simulink model "p2c1"  (R2023b)
settings: Solver=VariableStepAuto  StartTime=0.0  StopTime=100  RelTol=1e-3
settings Model: Creator=tanvi  LastModifiedBy=tanvi

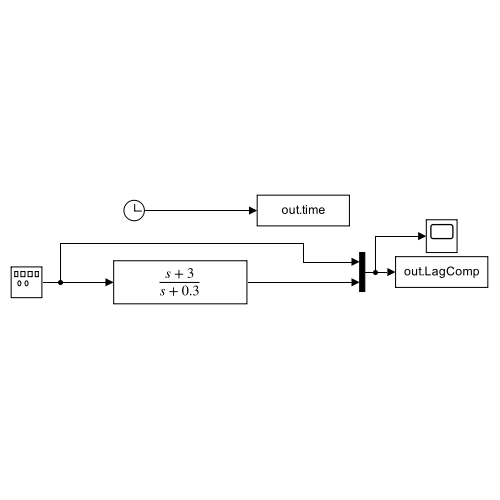
[thumbnail: Simulink's stored preview of the top-level diagram]
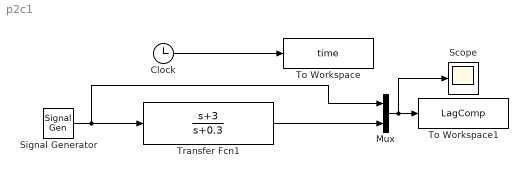
== system p2c1 ==
  Clock : Clock
  Mux : Mux  Inputs=2
  Scope : Scope
  Signal Generator : SignalGenerator  WaveForm=square  Frequency=0.02
  To Workspace : ToWorkspace  VariableName=time  SampleTime=-1
  To Workspace1 : ToWorkspace  VariableName=LagComp  SampleTime=-1
  Transfer Fcn1 : TransferFcn  Numerator=[1 3]  Denominator=[1 0.3]
  wires:
  Clock/1 -> To Workspace/1
  Signal Generator/1 -> Mux/1, Transfer Fcn1/1
  Transfer Fcn1/1 -> Mux/2
  Mux/1 -> Scope/1, To Workspace1/1
